simulink model "sim1link_base"  (R2025a)
settings: Solver=ode15s  StartTime=0.0  StopTime=10  RelTol=1e-3
undefined symbols (not defined in the file or in its folder): k
settings Model: Creator=yang  LastModifiedBy=yang

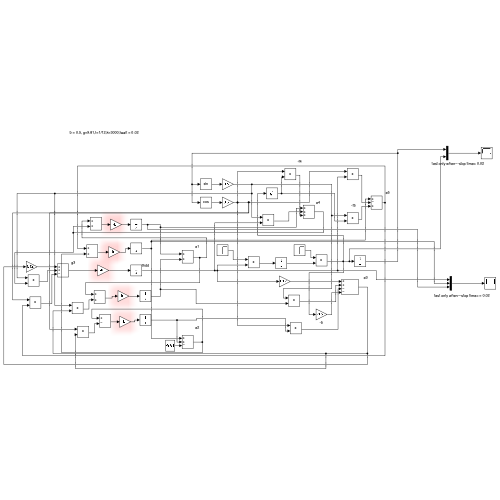
[thumbnail: Simulink's stored preview of the top-level diagram]
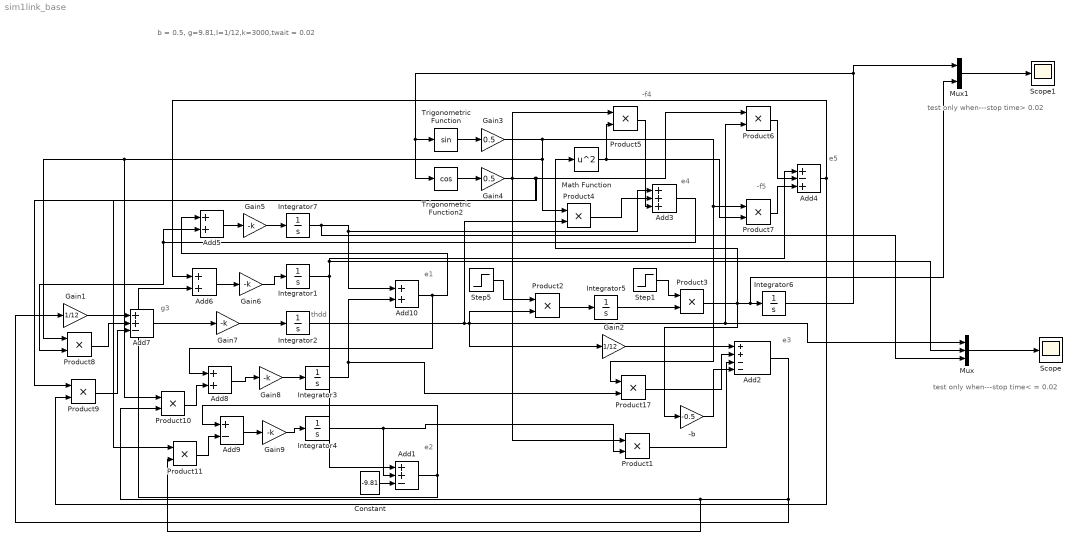
== system sim1link_base ==
  note: b = 0.5, g=9.81,I=1/12,k=3000,twait = 0.02
  note: test only when---stop time> 0.02
  note: test only when---stop time< = 0.02
  note: g3
  note: thdd
  note: e5
  note: -f5
  note: e4
  note: -f4
  note: e3
  note: e2
  note: e1
  -b : Gain  Gain=-0.5
  Add1 : Sum  Inputs=++-
  Add{5..6,8,10} (4 alike) : Sum
  Add2 : Sum  Inputs=++--
  Add3 : Sum  Inputs=+++
  Add4 : Sum  Inputs=+-+
  Add7 : Sum  Inputs=++-
  Add9 : Sum  Inputs=+-
  Constant : Constant  Value=-9.81
  Gain1 : Gain  Gain=1/12
  Gain2 : Gain  Gain=1/12
  Gain3 : Gain  Gain=0.5
  Gain4 : Gain  Gain=0.5
  Gain{5..9} (5 alike) : Gain  Gain=-k
  Integrator{1..7} (7 alike) : Integrator
  Math Function : Math  Operator=square
  Mux : Mux  Inputs=3
  Mux1 : Mux  Inputs=2
  Product{1..11,17} (12 alike) : Product
  Scope : Scope
      settings: ActiveDisplayYMinimum=-5.0200349208924635  ActiveDisplayYMaximum=11.640131295699405
  Scope1 : Scope
      settings: ActiveDisplayYMinimum=-4.8678600153474365  ActiveDisplayYMaximum=3.0296242559161675
  Step1 : Step  Time=0.02  SampleTime=0
  Step5 : Step  Time=0.02  SampleTime=0
  Trigonometric Function : Trigonometry
  Trigonometric Function2 : Trigonometry  Operator=cos
  wires:
  Trigonometric Function/1 -> Gain3/1
  Trigonometric Function2/1 -> Gain4/1
  Integrator3/1 -> Product17/2, Add10/2
  Integrator1/1 -> Mux/2, Add4/1, Add1/1
  Integrator4/1 -> Product1/2, Add1/2
  Constant/1 -> Add1/3
  Integrator2/1 -> Mux/1, Product6/2, Product2/2, Gain2/1, Product4/2
  Gain2/1 -> Add2/1
  Gain3/1 -> Product10/1, Product8/1, Product4/1, Product7/1, Product17/1
  Product17/1 -> Add2/2
  Gain4/1 -> Product11/1, Product9/1, Product6/1, Product5/1, Product1/1
  Product1/1 -> Add2/3
  Step5/1 -> Product2/1
  Product2/1 -> Integrator5/1
  Step1/1 -> Product3/1
  Integrator5/1 -> Product3/2
  -b/1 -> Add2/4
  Product3/1 -> Math Function/1, -b/1, Mux1/2, Integrator6/1
  Integrator7/1 -> Mux/3, Add3/1, Add10/1
  Product4/1 -> Add3/2
  Math Function/1 -> Product5/2, Product7/2
  Product5/1 -> Add3/3
  Product6/1 -> Add4/2
  Product7/1 -> Add4/3
  Add10/1 -> Add8/1, Add5/1
  Add3/1 -> Product8/2, Add5/2
  Add1/1 -> Add9/1, Add6/2
  Add4/1 -> Add6/1, Product9/2
  Add2/1 -> Product11/2, Product10/2, Gain1/1
  Gain1/1 -> Add7/1
  Product8/1 -> Add7/2
  Product9/1 -> Add7/3
  Product10/1 -> Add8/2
  Product11/1 -> Add9/2
  Mux/1 -> Scope/1
  Add5/1 -> Gain5/1
  Gain5/1 -> Integrator7/1
  Add6/1 -> Gain6/1
  Gain6/1 -> Integrator1/1
  Add7/1 -> Gain7/1
  Gain7/1 -> Integrator2/1
  Gain8/1 -> Integrator3/1
  Add8/1 -> Gain8/1
  Add9/1 -> Gain9/1
  Gain9/1 -> Integrator4/1
  Mux1/1 -> Scope1/1
  Integrator6/1 -> Mux1/1, Trigonometric Function2/1, Trigonometric Function/1
